simulink model "DCMotSimu"  (R2025a)
settings: Solver=VariableStepAuto  StartTime=0.0  StopTime=10.0  RelTol=1e-3
values from neighbouring files (symbols this model uses):
  B = 0.01    [DCMotPara.m]
  KePhi = 1.6    [DCMotPara.m]
  Ra = 0.5    [DCMotPara.m]
  tau_a = La/Ra    (= 0.2)    [DCMotPara.m]
  tau_m = J/B    (= 500)    [DCMotPara.m]
  TL = 50    [DCMotPara.m]
  Va = 160    [DCMotPara.m]
libraries: spspowerguiLib x1
settings Model: Creator=emilj  LastModifiedBy=emilj

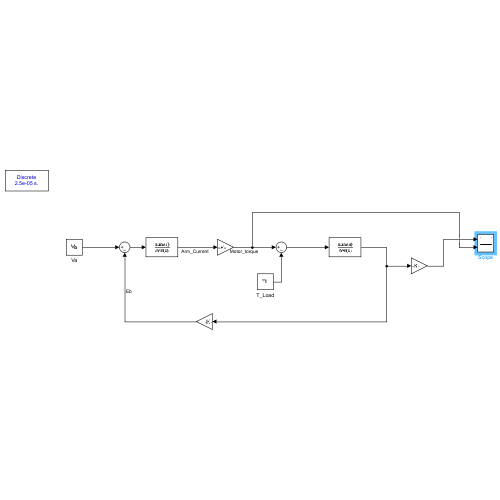
[thumbnail: Simulink's stored preview of the top-level diagram]
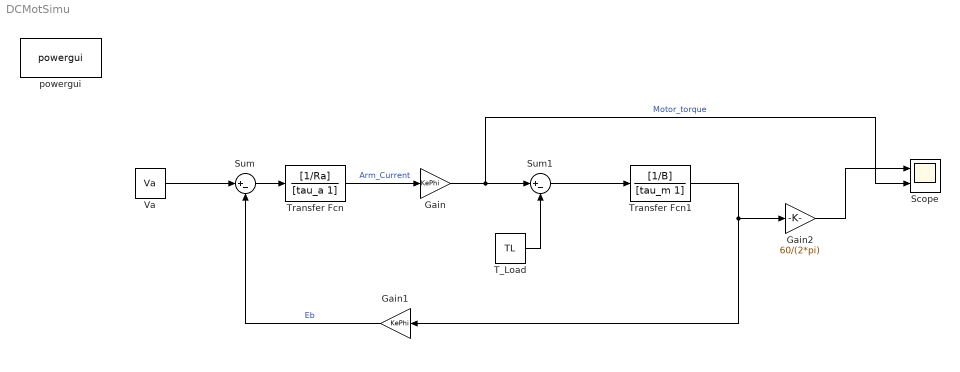
== system DCMotSimu ==
  Gain : Gain  Gain=KePhi
  Gain1 : Gain  Gain=KePhi
  Gain2 : Gain  Gain=60/(2*pi)
  Scope : Scope  NumInputPorts=2
      settings: Title=Torque  ActiveDisplayYMinimum=50.02894325891279  ActiveDisplayYMaximum=500.78644718809193  YLabel=Nm
  Sum : Sum  Inputs=|+-
  Sum1 : Sum  Inputs=|+-
  T_Load : Constant  Value=TL
  Transfer Fcn : TransferFcn  Numerator=[1/Ra]  Denominator=[tau_a 1]
  Transfer Fcn1 : TransferFcn  Numerator=[1/B]  Denominator=[tau_m 1]
  Va : Constant  Value=Va
  powergui : spspowerguiLib/powergui  Priority=1  SimulationMode=Discrete  SampleTime=25e-6  frequency=60  Iterations=50  frequencyindice=60  Pbase=100e6  ErrMax=1e-4  UnitsV=kV  UnitsW=MW  buscounter=0  FunctionMessages=off  echomessages=off  EnableUseOfTLC=off  CurrentSourceSwitches=off  DisableSnubberDevices=off  DisableRonSwitches=off  DisableVfSwitches=off  DisplayEquations=off  AutomaticDiscreteSolvers=off  SolverType=Tustin/Backward Euler (TBE)  Interpol=off  ExternalGateDelay=off  methode=off  Ts=100  x0status=blocks  SPID=on  SwTol=0  HookPort=off  NonlinearTolerance=1e-4  nMaxIteration=100  ContinueOnMaxIteration=off  RestoreLinks=warning  ResistiveCurrentMeasurement=off  Frange=[0:2:500]  Ylog=off  Xlog=on  ShowGrid=off  save=off  variable=ZData  structure=0  ZoomFFT=off  StartTime=0.0  cycles=1  DisplayStyle=1  fundamental=60  FreqAxis=off  MaxFrequency=1000  frequencyindicesteady=1  RmsSteady=1  display=off
  wires:
  Va/1 -> Sum/1
  Sum/1 -> Transfer Fcn/1
  Transfer Fcn/1 -> Gain/1  "Arm_Current"
  Gain/1 -> Scope/2, Sum1/1  "Motor_torque"
  T_Load/1 -> Sum1/2
  Sum1/1 -> Transfer Fcn1/1
  Transfer Fcn1/1 -> Gain1/1, Gain2/1
  Gain1/1 -> Sum/2  "Eb"
  Gain2/1 -> Scope/1
